simulink model "Microgrid_transition_model_113021_ben"  (R2020a)
settings: Solver=VariableStepAuto  StartTime=0.0  StopTime=1  MaxStep=1e-4  RelTol=1e-3
PreLoadFcn:
  | %run('FC_microgrid_param.m')
  | %load('gen_grid_init.mat')
InitFcn:
  | %load myisoModel_init;
  | run('FC_microgrid_param.m')
  | tic
  | run('CARTinitFcn.m')
  | %caseNo = 2;
  | 
  | %if (caseNo == 1)
  | %set_param(['Isolated_grid_paper_model_022521/SignalGen'], 'ActiveScenario', 'PStep222kW');
  | %else
  | %set_param(['Isolated_grid_paper_model_022521/SignalGen'], 'ActiveScenario', 'QStep222kVAr');
  | 
  | %end;
StopFcn:
  | toc
undefined symbols (not defined in the file or in its folder): breakpoints1, breakpoints2, cc_kp, cp_table_data, ctrl, D1, Delta, DiscIntNeverNeededParam, DT, FC_BESS, FC_PV_FirstSolar, find_system, gcbh, libFC_BESS, libFC_PV, LowerLimit, magnitude, oversize, pll_ki, pll_kp, pq_ts, sps_rtmsupport, timer, ts, Ts, Ts_APC, Ts_Control, Ts_Power, UpperLimit
libraries: powerlib x152, powerlib_extras x100, simulink x95, powerlib_meascontrol x90, eePowerMeasurement x40, pi_ctrl x16, simulink_extras x12, sps_avr x7, spsDieselMotorModel x3, libFSArray x2, SignalEditorBlockLib x2, libLgBattery x1
(part 14 of 14)

== system Microgrid_transition_model_113021_ben/Wind Turbine Type 4/Control/Measurement and Transformation/Discrete 3-phase PLL-Driven Positive-Sequence Active & Reactive Power/Discrete 3-phase PLL-Driven Positive-Sequence Fundamental Value/Discrete Variable Frequency Mean value2/Discrete Variable Transport Delay ==
  In : Inport
  D : Inport  Port=2
  "S-Function " : S-Function  FunctionName=discreteVariableTransportDelay  Parameters=MaxDelay,Ts,InitialValue  SFunctionDeploymentMode=off  EnableBusSupport=off
  Out : Outport  VectorParamsAs1DForOutWhenUnconnected=off
  wires:
  "S-Function "/1 -> Out/1
  In/1 -> "S-Function "/1
  D/1 -> "S-Function "/2

== system Microgrid_transition_model_113021_ben/Wind Turbine Type 4/Control/Measurement and Transformation/Discrete 3-phase PLL-Driven Positive-Sequence Active & Reactive Power/Discrete 3-phase PLL-Driven Positive-Sequence Fundamental Value2/Discrete Variable Frequency Mean value1/Correction subsystem ==
  N : Inport
  F : Inport  Port=2
  In : Inport  Port=3
  Gain1 : Gain  Gain=0.5  SaturateOnIntegerOverflow=on  OutDataTypeStr=Inherit: Same as input  ParamDataTypeStr=Inherit: Same as input
  Product2 : Product  Inputs=*/  InputSameDT=on  SaturateOnIntegerOverflow=on  OutDataTypeStr=Inherit: Same as first input
  Product4 : Product  Inputs=**  InputSameDT=on  SaturateOnIntegerOverflow=on  OutDataTypeStr=Inherit: Same as first input
  Product5 : Product  Inputs=**  InputSameDT=on  SaturateOnIntegerOverflow=on  OutDataTypeStr=Inherit: Same as first input
  Sum1 : Sum  Inputs=+-  InputSameDT=on  SaturateOnIntegerOverflow=on  OutDataTypeStr=Inherit: Same as first input
  Sum4 : Sum  InputSameDT=on  SaturateOnIntegerOverflow=on  OutDataTypeStr=Inherit: Same as first input
  Sum5 : Sum  Inputs=+-  InputSameDT=on  SaturateOnIntegerOverflow=on  OutDataTypeStr=Inherit: Same as first input
  Unit Delay : UnitDelay  SampleTime=Ts  HasFrameUpgradeWarning=on
  Out : Outport  VectorParamsAs1DForOutWhenUnconnected=off
  wires:
  Unit Delay/1 -> Sum1/2
  N/1 -> Sum5/1, Product2/2
  F/1 -> Sum5/2
  Sum5/1 -> Product2/1, Product5/1
  Product2/1 -> Product4/1
  In/1 -> Sum1/1, Unit Delay/1, Sum4/2
  Sum1/1 -> Product5/2
  Product5/1 -> Gain1/1
  Gain1/1 -> Sum4/1
  Sum4/1 -> Product4/2
  Product4/1 -> Out/1

== system Microgrid_transition_model_113021_ben/Wind Turbine Type 4/Control/Measurement and Transformation/Discrete 3-phase PLL-Driven Positive-Sequence Active & Reactive Power/Discrete 3-phase PLL-Driven Positive-Sequence Fundamental Value2/Discrete Variable Frequency Mean value1/Discrete Variable Transport Delay ==
  In : Inport
  D : Inport  Port=2
  "S-Function " : S-Function  FunctionName=discreteVariableTransportDelay  Parameters=MaxDelay,Ts,InitialValue  SFunctionDeploymentMode=off  EnableBusSupport=off
  Out : Outport  VectorParamsAs1DForOutWhenUnconnected=off
  wires:
  "S-Function "/1 -> Out/1
  In/1 -> "S-Function "/1
  D/1 -> "S-Function "/2

== system Microgrid_transition_model_113021_ben/Wind Turbine Type 4/Control/Measurement and Transformation/Discrete 3-phase PLL-Driven Positive-Sequence Active & Reactive Power/Discrete 3-phase PLL-Driven Positive-Sequence Fundamental Value2/Discrete Variable Frequency Mean value2/Correction subsystem ==
  N : Inport
  F : Inport  Port=2
  In : Inport  Port=3
  Gain1 : Gain  Gain=0.5  SaturateOnIntegerOverflow=on  OutDataTypeStr=Inherit: Same as input  ParamDataTypeStr=Inherit: Same as input
  Product2 : Product  Inputs=*/  InputSameDT=on  SaturateOnIntegerOverflow=on  OutDataTypeStr=Inherit: Same as first input
  Product4 : Product  Inputs=**  InputSameDT=on  SaturateOnIntegerOverflow=on  OutDataTypeStr=Inherit: Same as first input
  Product5 : Product  Inputs=**  InputSameDT=on  SaturateOnIntegerOverflow=on  OutDataTypeStr=Inherit: Same as first input
  Sum1 : Sum  Inputs=+-  InputSameDT=on  SaturateOnIntegerOverflow=on  OutDataTypeStr=Inherit: Same as first input
  Sum4 : Sum  InputSameDT=on  SaturateOnIntegerOverflow=on  OutDataTypeStr=Inherit: Same as first input
  Sum5 : Sum  Inputs=+-  InputSameDT=on  SaturateOnIntegerOverflow=on  OutDataTypeStr=Inherit: Same as first input
  Unit Delay : UnitDelay  SampleTime=Ts  HasFrameUpgradeWarning=on
  Out : Outport  VectorParamsAs1DForOutWhenUnconnected=off
  wires:
  Product4/1 -> Out/1
  Sum4/1 -> Product4/2
  Gain1/1 -> Sum4/1
  Product5/1 -> Gain1/1
  Sum1/1 -> Product5/2
  In/1 -> Sum4/2, Unit Delay/1, Sum1/1
  Product2/1 -> Product4/1
  Sum5/1 -> Product5/1, Product2/1
  F/1 -> Sum5/2
  N/1 -> Product2/2, Sum5/1
  Unit Delay/1 -> Sum1/2

== system Microgrid_transition_model_113021_ben/Wind Turbine Type 4/Control/Measurement and Transformation/Discrete 3-phase PLL-Driven Positive-Sequence Active & Reactive Power/Discrete 3-phase PLL-Driven Positive-Sequence Fundamental Value2/Discrete Variable Frequency Mean value2/Discrete Variable Transport Delay ==
  In : Inport
  D : Inport  Port=2
  "S-Function " : S-Function  FunctionName=discreteVariableTransportDelay  Parameters=MaxDelay,Ts,InitialValue  SFunctionDeploymentMode=off  EnableBusSupport=off
  Out : Outport  VectorParamsAs1DForOutWhenUnconnected=off
  wires:
  D/1 -> "S-Function "/2
  In/1 -> "S-Function "/1
  "S-Function "/1 -> Out/1

== matlab function Microgrid_transition_model_113021_ben/Grid Feeder Protective Relay/R25 - Sync Check v0.1/deadbus fcn ==
  data: Vbus input; y output; Vline input
% Copyright (c) 2016 Massachusetts Institute of Technology
% Permission is hereby granted, free of charge, to any person obtaining a copy of this
% software and associated documentation files (the "Software"), to deal in the Software
% without restriction, including without limitation the rights to use, copy, modify,
% merge, publish, distribute, sublicense, and/or sell copies of the Software, and to
% permit persons to whom the Software is furnished to do so, subject to the following
% conditions:
%
%
% The above copyright notice and this permission notice shall be included in
% all copies or substantial portions of the Software.
%
% THE SOFTWARE IS PROVIDED "AS IS", WITHOUT WARRANTY OF ANY KIND, EXPRESS OR IMPLIED,
% INCLUDING BUT NOT LIMITED TO THE WARRANTIES OF MERCHANTABILITY, FITNESS FOR A
% PARTICULAR PURPOSE AND NONINFRINGEMENT. IN NO EVENT SHALL THE AUTHORS OR COPYRIGHT
% HOLDERS BE LIABLE FOR ANY CLAIM, DAMAGES OR OTHER LIABILITY, WHETHER IN AN ACTION
% OF CONTRACT, TORT OR OTHERWISE, ARISING FROM, OUT OF OR IN CONNECTION WITH THE
% SOFTWARE OR THE USE OR OTHER DEALINGS IN THE SOFTWARE.
%
%
%%

function y = fcn(Vbus, Vline)
%#codegen
if isnan(Vbus)
    Vbus=0;
elseif isnan(Vline)
    Vline = 0;
end

% voltage threshold for deadbus
threshold = 0.05; % @ 5%

% bounding open-circuit voltage at 120%
a = (Vbus>(0.8)) && (Vbus<1.20) && (Vline < threshold);
b = (Vline>(0.8)) && (Vline<1.20) && (Vbus < threshold);
c = (Vline<threshold) && (Vbus < threshold);
y = a||b||c;

== matlab function Microgrid_transition_model_113021_ben/FC_PV_FirstSolar/MPPT Controller using Perturbe & Observe technique  ==
  settings: updateMethod=DISCRETE  sampleTime=Ts_Control
  data: Param input; Enabled input; V input; I input; D output
function D  = PandO(Param, Enabled, V, I)

% MPPT controller based on the Perturb & Observe algorithm.

% D output = Reference for DC link voltage (Vdc_ref) 
%
% Enabled input = 1 to enable the MPPT controller
% V input = PV array terminal voltage (V)
% I input = PV array current (A)
%
% Param input:
Dinit = Param(1);  %Initial value for Vdc_ref
Dmax = Param(2);   %Maximum value for Vdc_ref
Dmin = Param(3);   %Minimum value for Vdc_ref
deltaD = Param(4); %Increment value used to increase/decrease Vdc_ref
%  

persistent Vold Pold Dold;

dataType = 'double';

if isempty(Vold)
    Vold=0;
    Pold=0;
    Dold=Dinit;
end
P= V*I;
dV= V - Vold;
dP= P - Pold;

if dP ~= 0 & Enabled ~=0
    if dP < 0
        if dV < 0
            D = Dold + deltaD;
        else
            D = Dold - deltaD;
        end
    else
        if dV < 0
            D = Dold - deltaD;
        else
            D = Dold + deltaD;
        end    
    end
else D=Dold;
end

if D >= Dmax | D<= Dmin
    D=Dold;
end

Dold=D;
Vold=V;
Pold=P;

== matlab function Microgrid_transition_model_113021_ben/Wind Turbine Type 4/Fault Controller (atomic) /turbine_safety  ==
  data: ctrl input Bus: ctrlBus; data input Bus: dataBus; ctrl output; timer input Bus: timerBus; timer output; faulty parameter; dt input
 function [ctrl, timer]   = turbine_safety(ctrl, data, timer, faulty, dt)
    % Fault adaptive controller. Checks various sensor readings, and
    % responds by entering the appropriate control mode, providing the
    % appropriate torque derate, and setting the appropriate timers.
          
    % if faulted, don't change anything 
    if ctrl.mode(4)+ctrl.mode(5)+ctrl.mode(6) == 0 %if not faulted
        ctrl.RP_prev = ctrl.mode(2); %0 if ctrl.cmd =0; 1 otherwise
        fields = fieldnames(faulty); %run warning logic for all faultys
        ctrl.mode = [0,0,0,0,0,0];
        for i=1:length(fields)
            ctrl.(fields{i}).state = 0;
            checkHandle = str2func(faulty.(fields{i}).checkFun); %check for warnings/faultys
            ctrl = checkHandle(data, ctrl);
            ctrl = setMode(ctrl, faulty, fields{i}); %set mode
        end
        [ctrl, timer] = setTimers(ctrl, timer, dt); %set timers and torque derate
        ctrl.modeValue = sum(ctrl.mode.*2.^linspace(0,5,6));
    else
        if ctrl.mode(6) == 1
            fprintf('EMERGENCY STOP')
        elseif ctrl.mode(5) == 1
            fprintf('OPEN LOOP NORMAL STOP')
        elseif ctrl.mode(4) == 1
            fprintf('NORMAL STOP')
        end

%     displays for testing
%         disp('ctrl.mode:')
%         disp(ctrl.mode)
%         disp('data:')
%         disp(data)
%         disp('timer:')
%         disp(timer)
%         fprintf('data = %1.0f\n', data);
%         fprintf('ctrl.Ttarget = %1.0f\n', ctrl.Ttarget);

    end

== matlab function Microgrid_transition_model_113021_ben/Wind Turbine Type 4/APC (atomic)1/Inertial Response (to df)/FBIC/adaptive FBIC1 ==
  data: F_de input; Delta_P output; F_dr input; Wi input; P_de output; P_dr output; Act input
function [Delta_P,P_de,P_dr] = FBIC(F_de,F_dr,Wi,Act)
%Releasible kinetic energy based method by Dr. Kang 
if Act>=0.5
    
    Wmax=1;
    Wmin=0.9;
    R0=0.05;
    K0=1/R0/(Wmax^2-Wmin^2);
    
    Ri=R0*(Wmax^2-Wmin^2)/(Wi^2-Wmin^2);
    Ki=K0*(Wi^2-Wmin^2);
    P_dr=-1/Ri*F_dr;
    P_de=-Ki*F_de;
    Delta_P=P_dr+P_de;
else
    P_dr=0;
    P_de=0;
    Delta_P=0;
end

== matlab function Microgrid_transition_model_113021_ben/Wind Turbine Type 4/APC (atomic)1/Inertial Response (to df)/TLIC/adaptive TLIC ==
  data: recharge input; trecharge input; tIR input; Delta_P output; Act input; Ts_APC parameter; recharge output; trecharge output; tIR output
function [Delta_P, recharge, trecharge, tIR] = TLIC(recharge, trecharge, tIR, Act, Ts_APC)
%If frequency dips below deadband, provide max torque until rotor
%decelerates to x%. Then resume normal operation

Pmax = 1.3; %max power 1.3 pu

if recharge
    trecharge = trecharge + Ts_APC;
    Delta_P = 0;
    tIR = 0;
    if trecharge > 15
        recharge = 0;
    end
else
    trecharge = 0;
    if Act > 0.5 
        if tIR <= 3
            Delta_P = Pmax-1;
            tIR = tIR + Ts_APC;
        else
            Delta_P = 0;
            tIR = 0;
            recharge = 1;
        end
    else
        Delta_P = 0;
        tIR = 0;
    end
end

== matlab function Microgrid_transition_model_113021_ben/Grid Feeder Protective Relay1/R25 - Sync Check v0.1/deadbus fcn ==
  data: Vbus input; y output; Vline input
% Copyright (c) 2016 Massachusetts Institute of Technology
% Permission is hereby granted, free of charge, to any person obtaining a copy of this
% software and associated documentation files (the "Software"), to deal in the Software
% without restriction, including without limitation the rights to use, copy, modify,
% merge, publish, distribute, sublicense, and/or sell copies of the Software, and to
% permit persons to whom the Software is furnished to do so, subject to the following
% conditions:
%
%
% The above copyright notice and this permission notice shall be included in
% all copies or substantial portions of the Software.
%
% THE SOFTWARE IS PROVIDED "AS IS", WITHOUT WARRANTY OF ANY KIND, EXPRESS OR IMPLIED,
% INCLUDING BUT NOT LIMITED TO THE WARRANTIES OF MERCHANTABILITY, FITNESS FOR A
% PARTICULAR PURPOSE AND NONINFRINGEMENT. IN NO EVENT SHALL THE AUTHORS OR COPYRIGHT
% HOLDERS BE LIABLE FOR ANY CLAIM, DAMAGES OR OTHER LIABILITY, WHETHER IN AN ACTION
% OF CONTRACT, TORT OR OTHERWISE, ARISING FROM, OUT OF OR IN CONNECTION WITH THE
% SOFTWARE OR THE USE OR OTHER DEALINGS IN THE SOFTWARE.
%
%
%%

function y = fcn(Vbus, Vline)
%#codegen
if isnan(Vbus)
    Vbus=0;
elseif isnan(Vline)
    Vline = 0;
end

% voltage threshold for deadbus
threshold = 0.05; % @ 5%

% bounding open-circuit voltage at 120%
a = (Vbus>(0.8)) && (Vbus<1.20) && (Vline < threshold);
b = (Vline>(0.8)) && (Vline<1.20) && (Vbus < threshold);
c = (Vline<threshold) && (Vbus < threshold);
y = a||b||c;
